simulink model "sf_change_detection"  (Simulink 7.6)
settings: Solver=FixedStepDiscrete  StartTime=0.0  StopTime=10.0  FixedStep=.1  RelTol=1e-3
libraries: simulink x1
settings Model: Creator=The MathWorks Inc.  ExtModeAutoUpdateStatusClock=off
settings SolverCC: InsertRTBMode=Auto
settings OptimizationCC: InitFltsAndDblsToZero=on
settings DebuggingCC: SignalResolutionControl=TryResolveAllWithWarning  SolverPrmCheckMsg=none  StrictBusMsg=Warning
settings SFSimCC: SFSimEnableDebug=off  SFSimOverflowDetection=off  SFSimEcho=off  SimParseCustomCode=off
settings GRTTargetCC: TargetFcnLib=ansi_tfl_tmw.mat

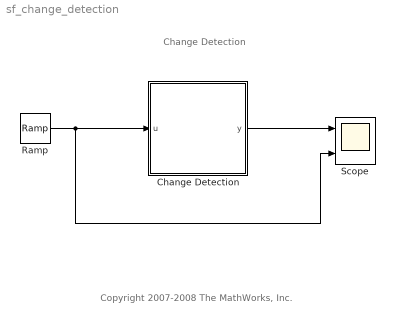
== system sf_change_detection ==
  note: Change Detection
  note: Copyright 2007-2008 The MathWorks, Inc.
  Change Detection : Stateflow chart  TreatAsAtomicUnit=on
  Ramp : simulink/Sources/Ramp  SystemSampleTime=-1  slope=1  start=0  X0=0
  Scope : Scope  NumInputPorts=2
      settings: YMin=-5~-5  YMax=5~5
  wires:
  Ramp/1 -> Change Detection/1(u), Scope/2
  Change Detection/1(y) -> Scope/1

== stateflow chart Change Detection ==
  state A
    y = 0;
  state B
    y = 1;
  state C
    du:
    y++;
  state D
    y = 3;
    du:
    x++;
  A -> B : [hasChanged(u)]
  B -> C : [hasChangedFrom(u,3)]
  C -> D : [hasChangedTo(y,10)]
  D -> A : [hasChangedFrom(x,3)]
  (default) -> A
  data: u input double; y output double; x local double
